simulink model "umts211_real"  (R2023b)
settings: Solver=VariableStepDiscrete  StartTime=0.0  StopTime=(N-1)*ts  RelTol=1e-3  EnableMultiTasking=on
values from neighbouring files (symbols this model uses):
  f = sort(f, 'descend')    [p1.m]    (also in sim211CascadeSDM_V2.m)
  fs = fs(valid_osr_idx)    [p1.m]    (also in sim211CascadeSDM_V2.m)
  gm1 = reshape(arrayfun(@(obj) obj.Variables(5).Value, SDin), [], 1)    [p1.m]    (also in sim211CascadeSDM_V2.m = gm1(valid_idx))
  gm2 = reshape(arrayfun(@(obj) obj.Variables(8).Value, SDin), [], 1)    [p1.m]    (also in sim211CascadeSDM_V2.m = gm2(valid_idx))
  gm3 = reshape(arrayfun(@(obj) obj.Variables(11).Value, SDin), [], 1)    [p1.m]    (also in sim211CascadeSDM_V2.m = gm3(valid_idx))
  gm4 = reshape(arrayfun(@(obj) obj.Variables(14).Value, SDin), [], 1)    [p1.m]    (also in sim211CascadeSDM_V2.m = gm4(valid_idx))
  ts = 1./fs    [p1.m]    (also in sim211CascadeSDM_V2.m)
undefined symbols (not defined in the file or in its folder): Adc1, Adc2, Adc3, Adc4, Ain, Avnl1, Avnl2, ci1, ci2, ci3, ci4, cl, cnl1, cnl2, cp1, cp2, cs1, cs2a, cs2b, cs3a, cs3b, cs4a, cs4b, FH, fin, FL, Io1, Io2, Io3, Io4, M, N, Ron, sinker, T, vosp, Vr
libraries: fesclib x4, quantidlib x3, simulink x2, dtoarealib x1
settings Model: Creator=rocio  LastModifiedBy=pmanrique
settings SolverCC: AlgebraicLoopSolver=TrustRegion
settings DataIOCC: LimitDataPoints=on  SaveFormat=Array  SignalLoggingSaveFormat=ModelDataLogs  ReturnWorkspaceOutputs=off
settings OptimizationCC: ExpressionDepthLimit=2147483647  InitFltsAndDblsToZero=on  LifeSpan=inf
settings DebuggingCC: SaveWithParameterizedLinksMsg=none  UnderspecifiedInitializationDetection=Classic  MergeDetectMultiDrivingBlocksExec=none  SignalResolutionControl=TryResolveAllWithWarning  SolverPrmCheckMsg=warning  MultiTaskDSMMsg=warning  MultiTaskCondExecSysMsg=none  FcnCallInpInsideContextMsg=warning  UnconnectedInputMsg=warning  UnconnectedOutputMsg=warning  UnconnectedLineMsg=warning  StateNameClashWarn=warning  SFUnexpectedBacktrackingDiag=warning  SFNoUnconditionalDefaultTransitionDiag=warning  SFExecutionAtInitializationDiag=none  ArithmeticOperatorsInVariantConditions=warning
settings HardwareCC: ProdBitPerPointer=32  ProdBitPerSizeT=32  ProdBitPerPtrDiffT=32  ProdLargestAtomicFloat=None  ProdIntDivRoundTo=Undefined  ProdEndianess=Unspecified  ProdWordSize=32  ProdHWDeviceType=32-bit Generic
settings ModelReferenceCC: PropagateSignalLabelsOutOfModel=off
settings SFSimCC: SimUseLocalCustomCode=off  CustomCodeUndefinedFunction=UseInterfaceOnly
settings RTWCC: RTWUseLocalCustomCode=off
settings CodeAppCC: StateflowObjectComments=on
settings GRTTargetCC: TargetFcnLib=ansi_tfl_tmw.mat  TargetLangStandard=C89/C90 (ANSI)  CombineOutputUpdateFcns=off  GRTInterface=on
settings ConfigComp: CovMetricSettings=dw  CovSaveCumulativeToWorkspaceVar=on  CovSaveSingleToWorkspaceVar=on  CovExternalEMLEnable=off

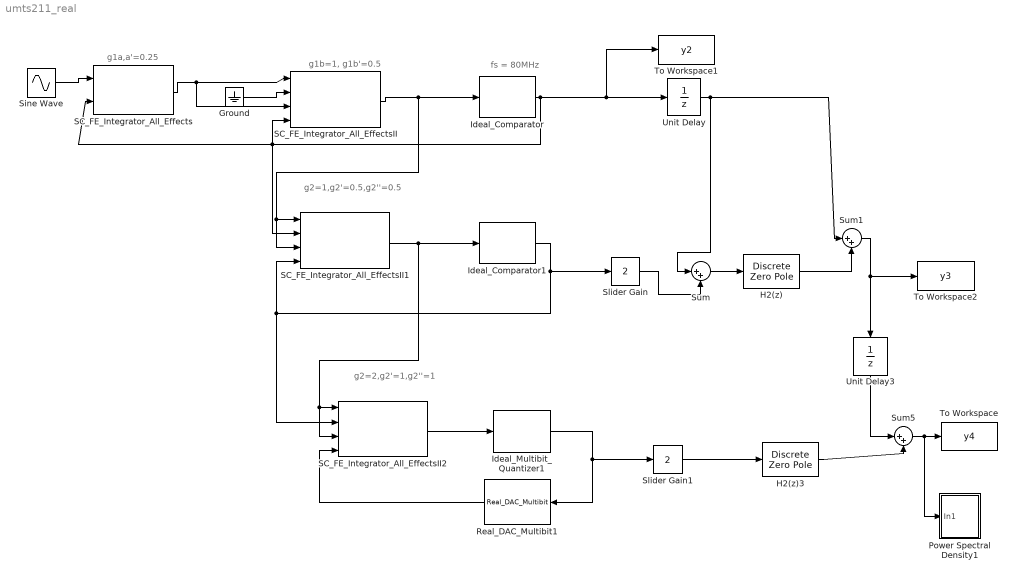
== system umts211_real ==
  note: g1a,a'=0.25
  note: g1b=1, g1b'=0.5
  note: g2=1,g2'=0.5,g2''=0.5
  note: g2=2,g2'=1,g2''=1
  note: fs = 80MHz
  Ground : Ground
  H2(z) : DiscreteZeroPole  Zeros=[1 1]  Poles=[0 0]  Gain=1  SampleTime=ts
  H2(z)3 : DiscreteZeroPole  Zeros=[1 1 1]  Poles=[0 0 0]  Gain=1  SampleTime=ts
  Ideal_Comparator : quantidlib/Ideal_Comparator  Vhigh=vhigh  Vlow=vlow  phi=phi1  ts=ts  qid=cuant1U
      link override Goto: GotoTag=cuant1U
  Ideal_Comparator1 : quantidlib/Ideal_Comparator  Vhigh=vhigh  Vlow=vlow  phi=phi1  ts=ts  qid=cuant2U
      link override Goto: GotoTag=cuant2U
  Ideal_Multibit_Quantizer1 : quantidlib/Ideal_Multibit_Quantizer  Vhigh=Vr  Vlow=-Vr  n_bits=B  Xfs=2*Vr  phi=phi1  ts=ts  qid=cuant3U
      link override Goto: GotoTag=cuant3U
  Power Spectral Density1 : Subsystem  AncestorBlock=SDtoolbox/Power Spectral Density  mask{SN=2, Fs=fs, fBL=1, fBH=fs/M, Fin=fin, N=N, Ntransient=0, VW=off, savename=savemat, Scale_type=linear}
      mask prompts: SN "Scope Number"; Fs "Sampling Frequency [Hz]"; fBL "Lower Band Bound [Hz]"; fBH "Upper Band Bound [Hz]"; Fin "Signal Frequency [Hz]"; N "Number of FFT Points"; Ntransient "Number of Transient Points"; VW "Variables Available in the Workspace"; savename "Nome of .mat File"; Scale_type "Scale"
      mask help: Calculates power spectral density, signal-to-noise ratio and effective number of bits of the Sigma-Delta modulator output
      mask init:
      | [f,FL,FH]=sinker_ini(Fs,fBL,fBH,Fin,N,SN);
      settings: LibrarySourceBlock=SDtoolbox/Power Spectral Density
      mask Help: web('PSD.html','-helpbrowser')
      mask Callback VW:
      | opt1=(get_param(gcb,'VW'));
      | switch opt1
      | 	case 'off'
      | 				set_param(gcb,'MaskEnables',{'on','on','on','on','on','on','on','on','off','on'});
      | 	case 'on'
      | 				set_param(gcb,'MaskEnables',{'on','on','on','on','on','on','on','on','on','on'});
      | end
      mask TypeOptions Scale_type: linear | logarithmic
      mask Display:
      | plot(0,0,1,1,[.14,.91,.91,.14,.14],[.86,.86,.40,.40,.86],[.85,.82,.80,.79,.75,.67,.63,.60,.57,.53,.41,.36,.33,.27,.24],[.49,.50,.53,.50,.49,.51,.54,.63,.54,.50,.50,.52,.82,.52,.45])
      | text(.54,.18, 'PSD','horizontalAlignment', 'center')
  Real_DAC_Multibit1 : dtoarealib/Real_DAC_Multibit  Vhigh=Vr  Vlow=-Vr  phi=phi1  ts=ts  n_bits=B  Xfs=2*Vr  inl_param=INL_LSB  gain_param=1  epsilong_param=0  epsilonoff_param=0
  SC_FE_Integrator_All_Effects : fesclib/SC_FE_Integrator_All_Effects  c=[cs1,ci1,cnl1,cnl2]  var=[0,0,T,Ron]  ops=[vosp,-vosp]  ao=[Adc1,gm1,Io1]  avnl=[Avnl1,Avnl2,0,0]  cp=[cp1,cp2,cl]  phi=phi1  ts=ts  settlingon=on  setin=on  idown=integ1  idnext=integ2
      link override Capacidades: Value=4e-13
      link override From: GotoTag=integ2
      link override Goto: GotoTag=integ1
  SC_FE_Integrator_All_EffectsII : fesclib/SC_FE_Integrator_All_EffectsII  c=[ci2,cs2a,cs2b,cnl1,cnl2]  var=[0,0,T,Ron]  ops=[vosp,-vosp]  ao=[Adc2,gm2,Io2]  avnl=[Avnl1,Avnl2,0,0]  cp=[cp1,cp2,cl]  phi=phi1  ts=ts  settlingon=on  setin=on  idown=integ2  idnext=integ3
      link override C11: Value=4e-13
      link override C12: Value=4e-13
      link override From: GotoTag=integ3
      link override Goto: GotoTag=integ2
  SC_FE_Integrator_All_EffectsII1 : fesclib/SC_FE_Integrator_All_EffectsII  c=[ci3,cs3a,cs3b,cnl1,cnl2]  var=[0,0,300,Ron]  ops=[vosp,-vosp]  ao=[Adc3,gm3,Io3]  avnl=[Avnl1,Avnl2,0,0]  cp=[cp1,cp2,cl]  phi=phi1  ts=ts  settlingon=on  setin=on  idown=integ3  idnext=integ4
      link override C11: Value=4e-13
      link override C12: Value=4e-13
      link override From: GotoTag=integ4
      link override Goto: GotoTag=integ3
  SC_FE_Integrator_All_EffectsII2 : fesclib/SC_FE_Integrator_All_EffectsII  c=[ci4,cs4a,cs4b,cnl1,cnl2]  var=[0,0,300,Ron]  ops=[vosp,-vosp]  ao=[Adc4,gm4,Io4]  avnl=[Avnl1,Avnl2,0,0]  cp=[cp1,cp2,cl]  phi=phi1  ts=ts  settlingon=on  setin=off  idown=integ4  idnext=integ4
      link override C11: Value=4e-13
      link override C12: Value=4e-13
      link override From: GotoTag=integ4
      link override Goto: GotoTag=integ4
  Sine Wave : Sin  Amplitude=Ain  Frequency=2*pi*fin  SampleTime=0
  Slider Gain : simulink/Math Operations/Slider Gain  gain=2  low=0  high=2
  Slider Gain1 : simulink/Math Operations/Slider Gain  gain=2  low=0  high=2
  Sum : Sum  Inputs=|++  SaturateOnIntegerOverflow=on
  Sum1 : Sum  Inputs=|++  SaturateOnIntegerOverflow=on
  Sum5 : Sum  Inputs=|++  SaturateOnIntegerOverflow=on
  To Workspace : ToWorkspace  VariableName=y4  SampleTime=ts
  To Workspace1 : ToWorkspace  VariableName=y2  SampleTime=ts
  To Workspace2 : ToWorkspace  VariableName=y3  SampleTime=ts
  Unit Delay : UnitDelay  SampleTime=ts
  Unit Delay3 : UnitDelay  SampleTime=ts
  wires:
  SC_FE_Integrator_All_EffectsII/1 -> Ideal_Comparator/1, SC_FE_Integrator_All_EffectsII1/3, SC_FE_Integrator_All_EffectsII1/1
  Ground/1 -> SC_FE_Integrator_All_EffectsII/2
  SC_FE_Integrator_All_Effects/1 -> SC_FE_Integrator_All_EffectsII/3, SC_FE_Integrator_All_EffectsII/1
  Sine Wave/1 -> SC_FE_Integrator_All_Effects/1
  Ideal_Comparator1/1 -> SC_FE_Integrator_All_EffectsII1/4, SC_FE_Integrator_All_EffectsII2/2, Slider Gain/1
  Ideal_Comparator/1 -> SC_FE_Integrator_All_Effects/2, SC_FE_Integrator_All_EffectsII/4, SC_FE_Integrator_All_EffectsII1/2, Unit Delay/1, To Workspace1/1
  Slider Gain/1 -> Sum/2
  Unit Delay/1 -> Sum1/1, Sum/1
  Sum/1 -> H2(z)/1
  SC_FE_Integrator_All_EffectsII1/1 -> SC_FE_Integrator_All_EffectsII2/3, SC_FE_Integrator_All_EffectsII2/1, Ideal_Comparator1/1
  H2(z)/1 -> Sum1/2
  Sum1/1 -> Unit Delay3/1, To Workspace2/1
  Ideal_Multibit_Quantizer1/1 -> Real_DAC_Multibit1/1, Slider Gain1/1
  SC_FE_Integrator_All_EffectsII2/1 -> Ideal_Multibit_Quantizer1/1
  Real_DAC_Multibit1/1 -> SC_FE_Integrator_All_EffectsII2/4
  Slider Gain1/1 -> H2(z)3/1
  Unit Delay3/1 -> Sum5/1
  H2(z)3/1 -> Sum5/2
  Sum5/1 -> Power Spectral Density1/1(In1), To Workspace/1

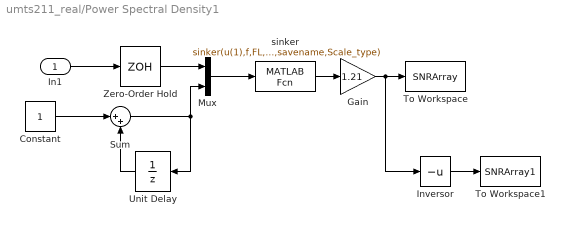
== system umts211_real/Power Spectral Density1 ==
  In1 : Inport
  Constant : Constant
  Gain : Gain  Gain=1.21
  Inversor : UnaryMinus
  Mux : Mux  Inputs=2
  Sum : Sum  Inputs=|++  SaturateOnIntegerOverflow=on
  To Workspace : ToWorkspace  VariableName=SNRArray  SampleTime=-1
      settings: MaxDataPoints=1
  To Workspace1 : ToWorkspace  VariableName=SNRArray1  SampleTime=-1
      settings: MaxDataPoints=1
  Unit Delay : UnitDelay  SampleTime=1/Fs  HasFrameUpgradeWarning=on
  Zero-Order Hold : ZeroOrderHold  SampleTime=1/Fs
  sinker : MATLABFcn  MATLABFcn=sinker(u(1),f,FL,FH,N,Ntransient,u(2),SN,Fs,VW,savename,Scale_type)
  wires:
  Zero-Order Hold/1 -> Mux/1
  In1/1 -> Zero-Order Hold/1
  Mux/1 -> sinker/1
  Sum/1 -> Mux/2, Unit Delay/1
  Constant/1 -> Sum/1
  Unit Delay/1 -> Sum/2
  sinker/1 -> Gain/1
  Inversor/1 -> To Workspace1/1
  Gain/1 -> To Workspace/1, Inversor/1
